simulink model "GMCLIB_PwmIct_BAM"  (Simulink 8.3)
settings: Solver=ode45  StartTime=0.0  StopTime=10.0  RelTol=1e-3
settings Model: Creator=nxa18952  LastModifiedBy=nxa18952
settings DataIOCC: SignalLoggingSaveFormat=Dataset
settings DebuggingCC: UnderspecifiedInitializationDetection=Simplified  StateNameClashWarn=none
settings GRTTargetCC: CombineOutputUpdateFcns=on  GRTInterface=off

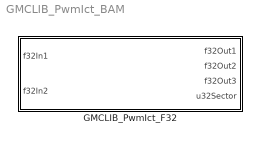
== system GMCLIB_PwmIct_BAM ==
  GMCLIB_PwmIct_F32 : Subsystem  mask(GMCLIB_PwmIct_F32){}
      mask help: Bit accurate model of General Sinusoidal PWM.
      mask init:
      | pos = get_param(gcb, 'Position');width = pos(3) - pos(1); height = pos(4) - pos(2);tX=width/2;tY=height*0.9;
      mask Display: color('black');port_label('input',1,'f32In1');port_label('input',2,'f32In2');port_label('output',1,'f32Out1');port_label('output',2,'f32Out2');port_label('output',3,'f32Out3');port_label('output',4,'u32Sector');color('black');disp('GMCLIB_PwmIct_F32');color('blue');text(tX,tY, 'BAM', 'horizontalAlignment', 'center');

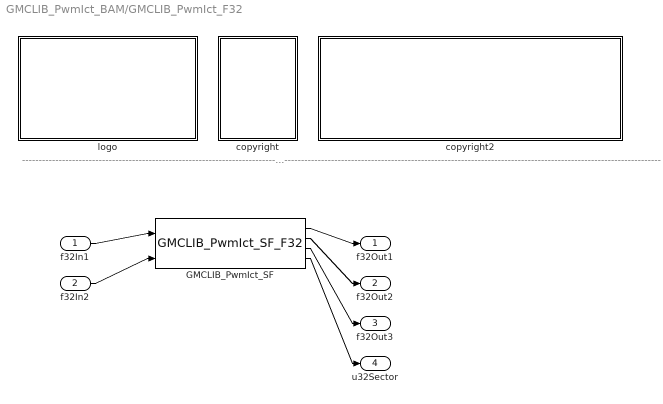
== system GMCLIB_PwmIct_BAM/GMCLIB_PwmIct_F32 ==
  note: ---------------------------------------------------------------------------------------------------------------------------------------------------------------------------------------------------
  f32In1 : Inport
  f32In2 : Inport  Port=2
  GMCLIB_PwmIct_SF : S-Function  FunctionName=GMCLIB_PwmIct_SF_F32  EnableBusSupport=off
  copyright : Subsystem
      mask Display: text(10,90,'FILE:');text(10,75,'DESRIPTION:');text(10,60,'COPYRIGHT:');text(10,45,'VERSION:');text(10,30,'DATE:')
  copyright2 : Subsystem
      mask Display: text(10,90,'GMCLIB_PwmIct_BAM_F32.mdl');text(10,75,'General Sinusoidal PWM.');text(10,60,'NXP');text(10,45,'1.0');text(10,30,'05-Apr-2019');
  logo : Subsystem
      mask Display: image(imread('logo.jpg'))
  f32Out1 : Outport
  f32Out2 : Outport  Port=2
  f32Out3 : Outport  Port=3
  u32Sector : Outport  Port=4
  wires:
  f32In1/1 -> GMCLIB_PwmIct_SF/1
  f32In2/1 -> GMCLIB_PwmIct_SF/2
  GMCLIB_PwmIct_SF/1 -> f32Out1/1
  GMCLIB_PwmIct_SF/2 -> f32Out2/1
  GMCLIB_PwmIct_SF/3 -> f32Out3/1
  GMCLIB_PwmIct_SF/4 -> u32Sector/1

== system GMCLIB_PwmIct_BAM/GMCLIB_PwmIct_F32/copyright ==

== system GMCLIB_PwmIct_BAM/GMCLIB_PwmIct_F32/copyright2 ==

== system GMCLIB_PwmIct_BAM/GMCLIB_PwmIct_F32/logo ==
